simulink library "etherlab_lib"  (R2017b)
(part 3 of 4)

      |                       hex2dec('8050'), hex2dec('0E'), sdo_8050_0E;
      |                       hex2dec('8050'), hex2dec('10'), sdo_8050_10;
      |                       hex2dec('8050'), hex2dec('12'), sdo_8050_12;
      |                       hex2dec('8050'), hex2dec('13'), sdo_8050_13;
      |                       hex2dec('8050'), hex2dec('14'), sdo_8050_14;
      |                       hex2dec('8050'), hex2dec('1E'), sdo_8050_1E;
      |                       hex2dec('8050'), hex2dec('1F'), sdo_8050_1F];
      | end
      | 
      | %save ep
      | rv = ep8309(model).configure(io);
      | 
      | EtherCATSlave.setPortNames(...
      |     {rv.PortConfig.input.portname},...
      |     {rv.PortConfig.output.portname});
      | 
      | set_param(gcb,'AttributesFormatString',...
      |     sprintf('%s\nM:%i Idx:%s',...
      |             model,master,mat2str(index)))
      settings: AttributesFormatString=|
      | EP8309-1022
      | M:0 Idx:1
      mask Help: web(etherlab_help_path('ep8309.html'), '-helpbrowser');
      mask TypeOptions model: EP8309-1022
      mask Callback model: ep8309().updateRevision()
      mask Callback anain: ep8309.updateAnalogIn
      mask TypeOptions sdo_F800_01: 0..20 mA | 4..20 mA
      mask TypeOptions sdo_F800_02: 0..20 mA | 4..20 mA
      mask TypeOptions sdo_8000_15: Off | 50Hz FIR | 60Hz FIR | IIR 1 | IIR 2 | IIR 3 | IIR 4 | IIR 5 | IIR 6 | IIR 7 | IIR 8
      mask TypeOptions tacho: None | Single shaft | Dual shaft
      mask Callback tacho: ep8309.updateTacho
      mask TypeOptions sdo_8020_15: RPM | 1/10 RPM | 1/100 RPM | Hz | 1/10 Hz | 1/100 Hz | 1/1000 Hz
      mask TypeOptions sdo_8030_15: RPM | 1/10 RPM | 1/100 RPM | Hz | 1/10 Hz | 1/100 Hz | 1/1000 Hz
      mask TypeOptions sdo_8031_15: RPM | 1/10 RPM | 1/100 RPM | Hz | 1/10 Hz | 1/100 Hz | 1/1000 Hz
      mask TypeOptions anaout: None | Current | PWM
      mask Callback anaout: ep8309.updateAnalogOut
      mask TypeOptions sdo_8050_05: Set to default | Ramp to default | Retain last value
      mask TypeOptions sdo_8060_05: Set to default | Ramp to default | Retain last value
      mask TypeOptions sdo_F800_08: 0..20 mA | 4..20 mA
      mask Display:
      | port_label('input', 1, 'DigOut')
      | port_label('output', 1, 'DigIn')
  Infrastructure : S-Function  LoadFcn=ekxxxx().checkModelName()  FunctionName=ec_slave3  Parameters=Address,rv.SlaveConfig,rv.PortConfig,debug,tsample  SFunctionModules='ecrt_support'  SFunctionDeploymentMode=off  EnableBusSupport=off  mask(EKxxxx){master=0, index=1, model=EK1100, revision=, vector=off, tsample=0, debug=0}
      mask prompts: index "Slave Index"; model "Device Model"; vector "Vector output"; tsample "Sample Time / Domain"
      mask help:
      | EtherCAT Infrastructure Slaves.
      |
      | Including these slaves (even if they don't have I/Os)
      | will create slave configurations, which will cause them to go into the
      | operational state.
      mask init:
      | Address = EtherCATSlave.formatAddress(master,index,tsample);
      | 
      | rv = ekxxxx(model).configure(vector);
      mask Help: web(etherlab_help_path('ekxxxx.html'), '-helpbrowser')
      mask TypeOptions model: EK1100 | EK1100-0030 | EK1101 | EK1110 | EK1122 | EK1200 | EK1501 | EK1501-0010 | EK1521 | EK1521-0010 | EK1541 | EK1561 | EK1814 | EK1818 | EK1828 | EK1828-0010 | CX1100-0004
      mask Callback model: ekxxxx().updateRevision()
      mask Display: fprintf('%s\nM:%i Idx:%s', model, master, mat2str(index))
